simulink model "Copy_of_FeedbackLinearizationController"  (R2019b)
settings: Solver=ode23t  StartTime=0.0  StopTime=25  RelTol=1e-3
undefined symbols (not defined in the file): B, b1, b2, C, D, gravity, Kd, Kp, l, q0, sigbuilder_block
settings Model: Creator=ariannagasparri  LastModifiedBy=ariannagasparri

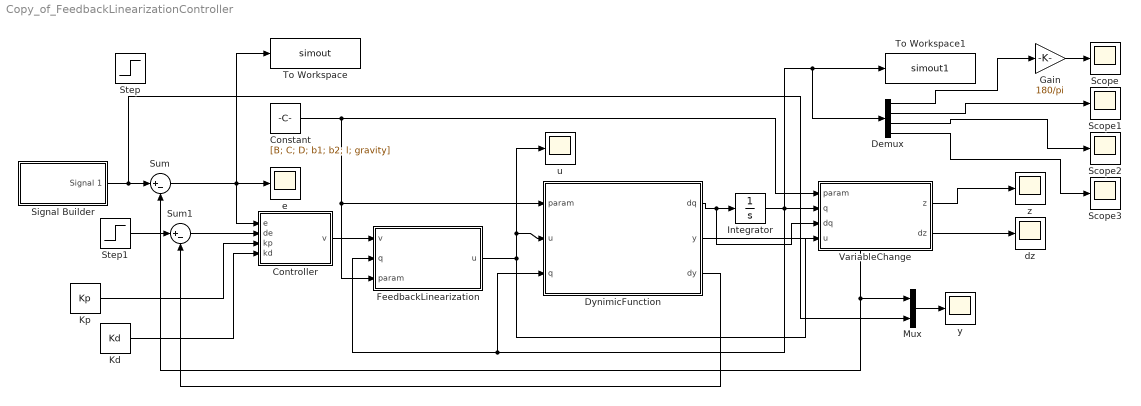
== system Copy_of_FeedbackLinearizationController ==
  Constant : Constant  Value=[B; C; D; b1; b2; l; gravity]
  Controller : MATLAB Function  TreatAsAtomicUnit=on
  Demux : Demux
  DynimicFunction : MATLAB Function  TreatAsAtomicUnit=on
  FeedbackLinearization : MATLAB Function  TreatAsAtomicUnit=on
  Gain : Gain  Gain=180/pi
  Integrator : Integrator  InitialCondition=q0
  Kd : Constant  Value=Kd
  Kp : Constant  Value=Kp
  Mux : Mux  Inputs=2
  Scope{,1..3} (4 alike) : Scope
  Signal Builder : Subsystem  Tag=STV Subsys  LoadFcn=sigbuilder_block('load',[437.6 199.2 550.4 400 ]);  StartFcn=sigbuilder_block('start');  StopFcn=sigbuilder_block('stop');  ClipboardFcn=sigbuilder_block('clipboard');  mask(Sigbuilder block){tuvar=[0:10]}
      mask help: Simulink:masks:SigbuilderBlock_MD
      mask init:
      | if ~strcmp(get_param(bdroot(gcbh),'SimulationStatus'),'stopped') tuvar = sigbuilder_block('maskInit'); end
      settings: CopyFcn=sigbuilder_block('copy');  DeleteFcn=sigbuilder_block('delete');  ModelCloseFcn=sigbuilder_block('modelClose');  PreSaveFcn=sigbuilder_block('preSave');  PauseFcn=sigbuilder_block('pause');  ContinueFcn=sigbuilder_block('continue');  NameChangeFcn=sigbuilder_block('namechange');  OpenFcn=sigbuilder_block('open',[437.6 199.2 550.4 400 ]);  CloseFcn=sigbuilder_block('close');
      mask Display: plot(0, 0, 100, 100,[2, 2, 32, 32, 2], [68, 8, 8, 68, 68],[32, 2], [38, 38], [32, 19, 2],[53, 60, 44], [32, 17, 17, 2],[16, 16, 31, 31]);txt = getActiveGroup(gcbh);text(2, 100, txt,'verticalAlignment', 'top');
  Step : Step  After=3+l*sin(0)  SampleTime=0
  Step1 : Step  After=0  SampleTime=0
  Sum : Sum  Inputs=|+-
  Sum1 : Sum  Inputs=|+-
  To Workspace : ToWorkspace  VariableName=simout  SaveFormat=Timeseries  SampleTime=-1
  To Workspace1 : ToWorkspace  VariableName=simout1  SaveFormat=Timeseries  SampleTime=-1
  VariableChange : MATLAB Function  TreatAsAtomicUnit=on
  dz : Scope
  e : Scope
  u : Scope
  y : Scope
  z : Scope
  wires:
  DynimicFunction/1(dq) -> VariableChange/3(dq), Integrator/1
  Sum/1 -> To Workspace/1, e/1, Controller/1(e)
  Constant/1 -> VariableChange/1(param), FeedbackLinearization/3(param), DynimicFunction/1(param)
  Signal Builder/1(Signal 1) -> Mux/2, Sum/1
  FeedbackLinearization/1(u) -> DynimicFunction/2(u), u/1, VariableChange/4(u)
  Controller/1(v) -> FeedbackLinearization/1(v)
  VariableChange/1(z) -> z/1
  Kp/1 -> Controller/3(kp)
  VariableChange/2(dz) -> dz/1
  Step1/1 -> Sum1/1
  DynimicFunction/2(y) -> Mux/1, Sum/2
  Kd/1 -> Controller/4(kd)
  Mux/1 -> y/1
  DynimicFunction/3(dy) -> Sum1/2
  Sum1/1 -> Controller/2(de)
  Demux/2 -> Scope1/1
  Integrator/1 -> Demux/1, To Workspace1/1, VariableChange/2(q), FeedbackLinearization/2(q), DynimicFunction/3(q)
  Demux/3 -> Scope2/1
  Demux/4 -> Scope3/1
  Gain/1 -> Scope/1
  Demux/1 -> Gain/1

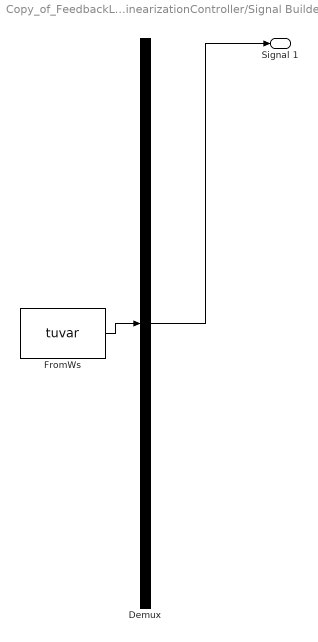
== system Copy_of_FeedbackLinearizationController/Signal Builder ==
  Demux : Demux  Tag=STV Demux  Outputs=1
  FromWs : FromWorkspace  Tag=STV FromWs  VariableName=tuvar  SampleTime=0
      SigBuilderData=|
      | common.afterFinalStr = 'Extrapolate'
      | common.sampleTime = 0
      | dataSet.timeRange = [0 10]
      | dataSet.name = 'Group 1'
      | sbobj.Groups.Name = 'Group 1'
      | sbobj.Groups.Signals.Name = 'Signal 1'
      | sbobj.Groups.Signals.XData = [0 0.5 1 10]
      | sbobj.Groups.Signals.YData = [0 0 3 3]
  Signal 1 : Outport  Tag=STV Outport
  wires:
  Demux/1 -> Signal 1/1
  FromWs/1 -> Demux/1

== matlab function Copy_of_FeedbackLinearizationController/FeedbackLinearization ==
  data: v input; u output; q input; param input
function u = FeedbackLinearization(v, q, param)

B = param(1);
C = param(2);
D = param(3);
b1 = param(4);
b2 = param(5);
l = param(6);
gravity = param(7);

u = (v - Lf2h_fun(B,C,D,b1,b2,gravity,l,q)) / LgLfh_fun(B,C,D,l,q);

end

== matlab function Copy_of_FeedbackLinearizationController/DynimicFunction ==
  data: param input; u input; dq output; q input; y output; dy output
function [dq, y, dy] = DynamicFunction(param, u, q)

B = param(1);
C = param(2);
D = param(3);
b1 = param(4);
b2 = param(5);
l = param(6);
gravity = param(7);

dq = f_fun(B,C,D,b1,b2,gravity,l,q) + g_fun(B,C,D,l,q)*u;
y = h_fun(l,q);
dy = dq(3) + l*cos(q(1))*dq(1);

end

== matlab function Copy_of_FeedbackLinearizationController/VariableChange ==
  data: param input; q input; dq input; z output; dz output; u input
function [z, dz] = VariableChange(param, q, dq, u)

z = zeros(4,1);
dz = zeros(4,1);

B = param(1);
C = param(2);
D = param(3);
b1 = param(4);
b2 = param(5);
l = param(6);
gravity = param(7);

z(1) = h_fun(l,q);
z(2) = Lfh_fun(l,q);
z(3) = q(1);
z(4) = (-1/(l*cos(q(1))*B))*q(2) + q(4);

dz(1) = z(2);
dz(2) = Lf2h_fun(B,C,D,b1,b2,gravity,l,q) + LgLfh_fun(B,C,D,l,q)*u;
dz(3) = dq(1);
dz(4) = u/(D*(C + B*l*cos(q(1)))) - (b2*q(4) + B*gravity*l*sin(q(1)))/(C + B*l*cos(q(1))) + ((b1*q(2))/D + (B*gravity*l*sin(q(1)))/D + (B*l*cos(q(1))*(b2*q(4) + B*gravity*l*sin(q(1))))/(D*(C + B*l*cos(q(1)))) + (B*u*l*cos(q(1)))/(D*(C + B*l*cos(q(1)))))/(B*l*cos(q(1))) - (q(2)^2*sin(q(1)))/(B*l*cos(q(1))^2);

end

== matlab function Copy_of_FeedbackLinearizationController/Controller ==
  data: e input; de input; v output; kp input; kd input
function v = Controller(e,de,kp,kd)

v = kp * e + kd * de;

end
